simulink model "UNCOMPENSATED_OP"  (R2025b)
settings: Solver=VariableStepAuto  StartTime=0.0  StopTime=0.01  RelTol=1e-3
values from neighbouring files (symbols this model uses):
  fsw = 200e3    (= 200000)    [CL_TF.m]    (also in Cullums_Digital_amp.m; Cullums_analog_amp.m; Integrator489.m; OP_TF_K.m)
  Glc = 1 / (L*C*s^2 + (L/R)*s + 1)    [CL_TF.m]    (also in Integrator489.m; OP_TF_K.m; OP_TF_TYPE1.m; OP_TF_Type2.m)
  Vc = 5    [CL_TF.m]    (also in Integrator489.m; OP_TF_K.m; OP_TF_TYPE1.m; OP_TF_Type2.m)
  Vtri = 1.6    [CL_TF.m]    (also in Integrator489.m; OP_TF_K.m; OP_TF_TYPE1.m; OP_TF_Type2.m)
libraries: simulink x1
settings Model: Creator=toumoucull  LastModifiedBy=toumoucull

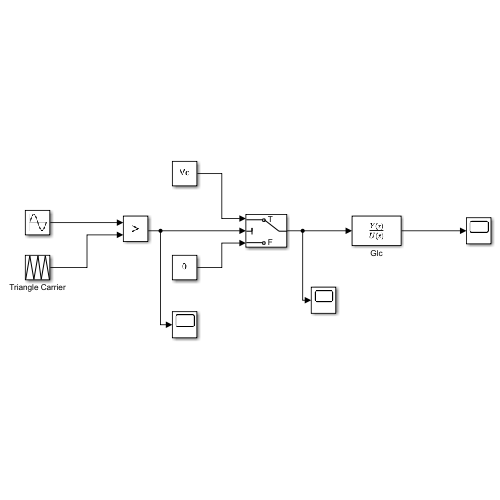
[thumbnail: Simulink's stored preview of the top-level diagram]
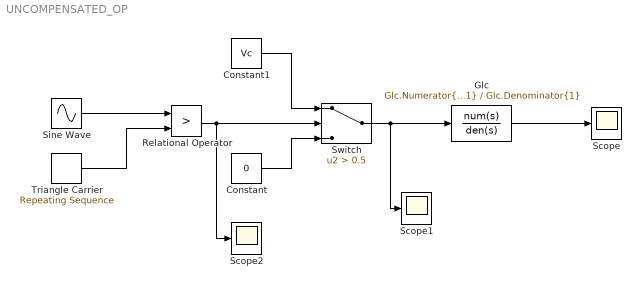
== system UNCOMPENSATED_OP ==
  Constant : Constant  Value=0
  Constant1 : Constant  Value=Vc
  Glc : TransferFcn  Numerator=Glc.Numerator{1}  Denominator=Glc.Denominator{1}
  Relational Operator : RelationalOperator  Operator=>  OutDataTypeStr=boolean  RndMeth=Simplest  InputSameDT=off
  Scope : Scope
      settings: ActiveDisplayYMinimum=-2.5618142036368665  ActiveDisplayYMaximum=7.1546514169373285
  Scope1 : Scope
      settings: ActiveDisplayYMinimum=-0.62499999999999989  ActiveDisplayYMaximum=5.625
  Scope2 : Scope
      settings: ActiveDisplayYMinimum=-0.12499999999999997  ActiveDisplayYMaximum=1.125  DataLoggingVariableName=ScopeData2
  Sine Wave : Sin  Frequency=2*pi*1000  SampleTime=0
  Switch : Switch  Criteria=u2 > Threshold  Threshold=0.5  SaturateOnIntegerOverflow=off  InputSameDT=off
  Triangle Carrier : simulink/Sources/Repeating Sequence  rep_seq_t=[0 1/(2*fsw) 1/fsw]  rep_seq_y=[-Vtri Vtri -Vtri]
  wires:
  Sine Wave/1 -> Relational Operator/1
  Triangle Carrier/1 -> Relational Operator/2
  Constant1/1 -> Switch/1
  Constant/1 -> Switch/3
  Relational Operator/1 -> Scope2/1, Switch/2
  Switch/1 -> Scope1/1, Glc/1
  Glc/1 -> Scope/1
